simulink model "sim_filterComplementary_measData_16b"  (R2016b)
settings: Solver=FixedStepAuto  StartTime=0.0  StopTime=30  FixedStep=1e-1  RelTol=1e-3
values from neighbouring files (symbols this model uses):
  w0 = w0s(ii)    [sim_filterComplementary_measData_init.m]
libraries: simulink x3
settings Model: Creator=Nu  LastModifiedBy=Nu

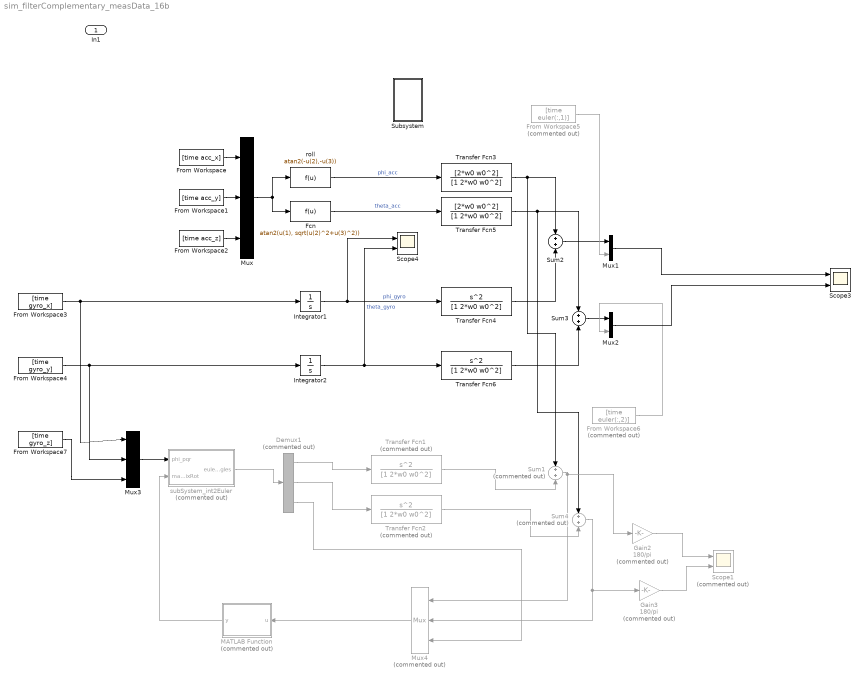
== system sim_filterComplementary_measData_16b ==
  In1 : Inport
  Demux1 : Demux  Commented=on  Outputs=3
  Fcn : Fcn  Expr=atan2(u(1), sqrt(u(2)^2+u(3)^2))
  From Workspace : FromWorkspace  VariableName=[time acc_x]  SampleTime=0
  From Workspace1 : FromWorkspace  VariableName=[time acc_y]  SampleTime=0
  From Workspace2 : FromWorkspace  VariableName=[time acc_z]  SampleTime=0
  From Workspace3 : FromWorkspace  VariableName=[time gyro_x]  SampleTime=0
  From Workspace4 : FromWorkspace  VariableName=[time gyro_y]  SampleTime=0
  From Workspace5 : FromWorkspace  Commented=on  VariableName=[time euler(:,1)]  SampleTime=0
  From Workspace6 : FromWorkspace  Commented=on  VariableName=[time euler(:,2)]  SampleTime=0
  From Workspace7 : FromWorkspace  VariableName=[time gyro_z]  SampleTime=0
  Gain2 : Gain  Commented=on  Gain=180/pi
  Gain3 : Gain  Commented=on  Gain=180/pi
  Integrator1 : Integrator
  Integrator2 : Integrator
  MATLAB Function : MATLAB Function  Commented=on  TreatAsAtomicUnit=on
  Mux : Mux  Inputs=3
  Mux1 : Mux  Inputs=2
  Mux2 : Mux  Inputs=2
  Mux3 : Mux  Inputs=3
  Mux4 : Mux  Commented=on  Inputs=3
  Scope1 : Scope  Commented=on  NumInputPorts=2
  Scope3 : Scope  NumInputPorts=2
  Scope4 : Scope  NumInputPorts=2
  Subsystem : Subsystem
  Sum1 : Sum  Commented=on
  Sum2 : Sum
  Sum3 : Sum
  Sum4 : Sum  Commented=on
  Transfer Fcn1 : TransferFcn  Commented=on  Numerator=[1 0 0]  Denominator=[1 2*w0 w0^2]
  Transfer Fcn2 : TransferFcn  Commented=on  Numerator=[1 0 0]  Denominator=[1 2*w0 w0^2]
  Transfer Fcn3 : TransferFcn  Numerator=[2*w0 w0^2]  Denominator=[1 2*w0 w0^2]
  Transfer Fcn4 : TransferFcn  Numerator=[1 0 0]  Denominator=[1 2*w0 w0^2]
  Transfer Fcn5 : TransferFcn  Numerator=[2*w0 w0^2]  Denominator=[1 2*w0 w0^2]
  Transfer Fcn6 : TransferFcn  Numerator=[1 0 0]  Denominator=[1 2*w0 w0^2]
  roll : Fcn  Expr=atan2(-u(2),-u(3))
  subSystem_int2Euler : Subsystem  Commented=on
  wires:
  From Workspace/1 -> Mux/1
  From Workspace1/1 -> Mux/2
  From Workspace2/1 -> Mux/3
  Mux/1 -> Fcn/1, roll/1
  roll/1 -> Transfer Fcn3/1  "phi_acc"
  From Workspace3/1 -> Mux3/1, Integrator1/1
  Integrator1/1 -> Scope4/1, Transfer Fcn4/1  "phi_gyro"
  Transfer Fcn3/1 -> Sum1/1, Sum2/1
  Transfer Fcn4/1 -> Sum2/2
  Fcn/1 -> Transfer Fcn5/1  "theta_acc"
  From Workspace4/1 -> Mux3/2, Integrator2/1
  Integrator2/1 -> Scope4/2, Transfer Fcn6/1  "theta_gyro"
  Transfer Fcn5/1 -> Sum4/1, Sum3/1
  Sum2/1 -> Mux1/1
  Transfer Fcn6/1 -> Sum3/2
  Sum3/1 -> Mux2/1
  From Workspace5/1 -> Mux1/2
  From Workspace6/1 -> Mux2/2
  Mux1/1 -> Scope3/1
  Mux2/1 -> Scope3/2
  Mux3/1 -> subSystem_int2Euler/1(phi_pqr)
  From Workspace7/1 -> Mux3/3
  subSystem_int2Euler/1(eulerAngles) -> Demux1/1
  Transfer Fcn1/1 -> Sum1/2
  Transfer Fcn2/1 -> Sum4/2
  Mux4/1 -> MATLAB Function/1(u)
  Sum1/1 -> Gain2/1, Mux4/1
  Sum4/1 -> Gain3/1, Mux4/2
  Demux1/3 -> Mux4/3
  MATLAB Function/1(y) -> subSystem_int2Euler/2(matrixRot)
  Gain2/1 -> Scope1/1
  Gain3/1 -> Scope1/2
  Demux1/1 -> Transfer Fcn1/1
  Demux1/2 -> Transfer Fcn2/1

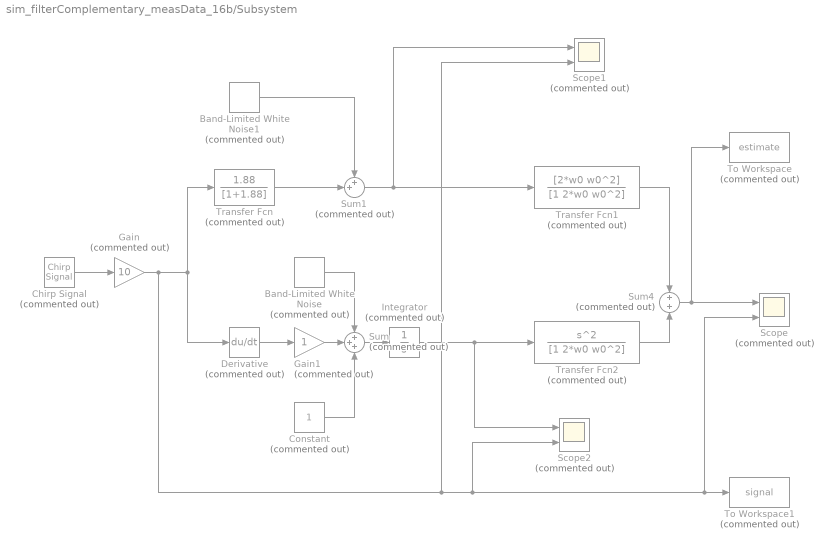
== system sim_filterComplementary_measData_16b/Subsystem ==
  Band-Limited White Noise : simulink/Sources/Band-Limited White Noise  Commented=on  Cov=[0.1]  Ts=0.1  seed=[23341]
  Band-Limited White Noise1 : simulink/Sources/Band-Limited White Noise  Commented=on  Cov=[0.1]  Ts=0.1  seed=[23341]
  Chirp Signal : simulink/Sources/Chirp Signal  Commented=on  f1=0.1  T=100  f2=0.05
  Constant : Constant  Commented=on
  Derivative : Derivative  Commented=on
  Gain : Gain  Commented=on  Gain=10
  Gain1 : Gain  Commented=on
  Integrator : Integrator  Commented=on
  Scope : Scope  Commented=on  NumInputPorts=2
  Scope1 : Scope  Commented=on  NumInputPorts=2
  Scope2 : Scope  Commented=on  NumInputPorts=2
  Sum : Sum  Commented=on  Inputs=+++
  Sum1 : Sum  Commented=on  Inputs=++|
  Sum4 : Sum  Commented=on
  To Workspace : ToWorkspace  Commented=on  VariableName=estimate  SampleTime=-1
  To Workspace1 : ToWorkspace  Commented=on  VariableName=signal  SampleTime=-1
  Transfer Fcn : TransferFcn  Commented=on  Numerator=[1.88]  Denominator=[1+1.88]
  Transfer Fcn1 : TransferFcn  Commented=on  Numerator=[2*w0 w0^2]  Denominator=[1 2*w0 w0^2]
  Transfer Fcn2 : TransferFcn  Commented=on  Numerator=[1 0 0]  Denominator=[1 2*w0 w0^2]
  wires:
  Chirp Signal/1 -> Gain/1
  Transfer Fcn/1 -> Sum1/2
  Transfer Fcn1/1 -> Sum4/1
  Transfer Fcn2/1 -> Sum4/2
  Band-Limited White Noise/1 -> Sum/1
  Constant/1 -> Sum/3
  Sum4/1 -> To Workspace/1, Scope/1
  Gain/1 -> Scope1/2, Scope2/2, Scope/2, To Workspace1/1, Transfer Fcn/1, Derivative/1
  Sum/1 -> Integrator/1
  Integrator/1 -> Scope2/1, Transfer Fcn2/1
  Sum1/1 -> Scope1/1, Transfer Fcn1/1
  Derivative/1 -> Gain1/1
  Gain1/1 -> Sum/2
  Band-Limited White Noise1/1 -> Sum1/1

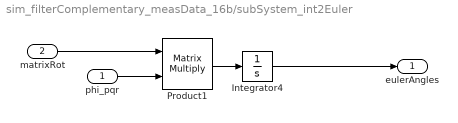
== system sim_filterComplementary_measData_16b/subSystem_int2Euler ==
  phi_pqr : Inport
  matrixRot : Inport  Port=2
  Integrator4 : Integrator  InitialCondition=zeros(3,1)
  Product1 : Product  Multiplication=Matrix(*)
  eulerAngles : Outport
  wires:
  Integrator4/1 -> eulerAngles/1
  Product1/1 -> Integrator4/1
  phi_pqr/1 -> Product1/2
  matrixRot/1 -> Product1/1

== matlab function sim_filterComplementary_measData_16b/MATLAB Function ==
  data: u input; y output
function y = fcn(u)
A = [cos(u(2)) 0 -cos(u(1))*sin(u(2));
     0 1 sin(u(1));
     sin(u(2)) 0 cos(u(1))*cos(u(2))];
y = A;
